simulink model "2293_2020_TP1_Parra_fgh"  (R2019b)
settings: Solver=ode45  StartTime=0.0  StopTime=10  FixedStep=0.001  RelTol=1e-3
undefined symbols (not defined in the file): A, B, C, ki, kp, L, ueq, xeq, yref
settings Model: Creator=aghersin  LastModifiedBy=rochi
settings DataIOCC: ReturnWorkspaceOutputs=off
settings DebuggingCC: ArithmeticOperatorsInVariantConditions=warning
settings SFSimCC: SimUseLocalCustomCode=off  CustomCodeUndefinedFunction=UseInterfaceOnly
settings RTWCC: RTWUseLocalCustomCode=off

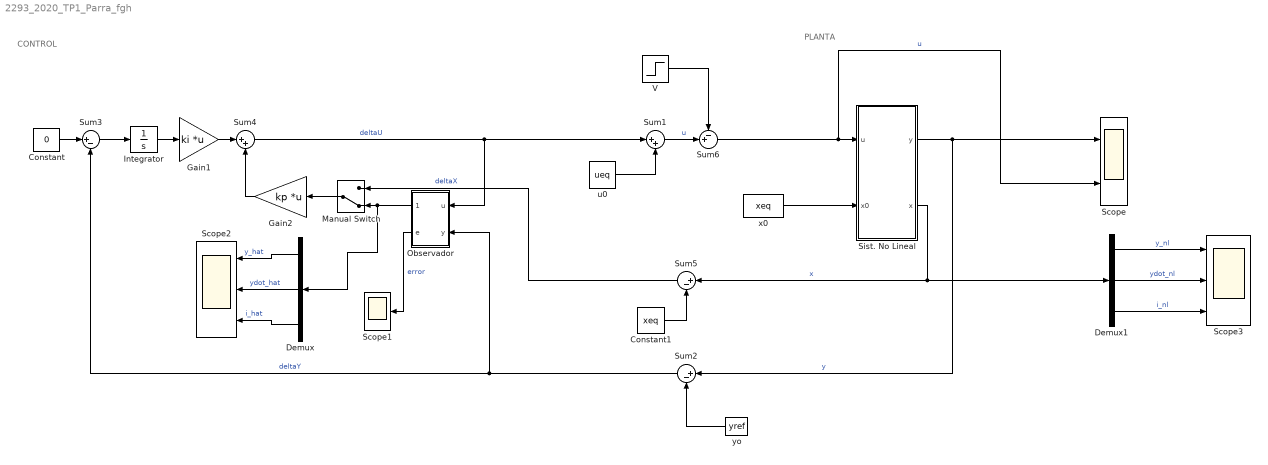
== system 2293_2020_TP1_Parra_fgh ==
  note: CONTROL
  note: PLANTA
  Constant : Constant  Value=0
  Constant1 : Constant  Value=xeq
  Demux : Demux  Outputs=3
  Demux1 : Demux  Outputs=3
  Gain1 : Gain  Gain=ki  Multiplication=Matrix(K*u)
  Gain2 : Gain  Gain=kp  Multiplication=Matrix(K*u)
  Integrator : Integrator
  Manual Switch : ManualSwitch  CurrentSetting=0
  Observador : Subsystem
  Scope : Scope  NumInputPorts=2
  Scope1 : Scope
  Scope2 : Scope  NumInputPorts=3
  Scope3 : Scope  NumInputPorts=3
  "Sist. No Lineal " : Subsystem
  Sum1 : Sum  Inputs=|++
  Sum2 : Sum  Inputs=|+-
  Sum3 : Sum  Inputs=|+-
  Sum4 : Sum  Inputs=|++
  Sum5 : Sum  Inputs=|+-
  Sum6 : Sum  Inputs=-+|
  V : Step  Time=5  SampleTime=0
  u0 : Constant  Value=ueq
  x0 : Constant  Value=xeq
  yo : Constant  Value=yref
  wires:
  Gain2/1 -> Sum4/2
  Sum4/1 -> Sum1/1, Observador/1(u)  "deltaU"
  Constant/1 -> Sum3/1
  Sum3/1 -> Integrator/1
  u0/1 -> Sum1/2
  Integrator/1 -> Gain1/1
  Sum1/1 -> Sum6/2  "u"
  Observador/2(e) -> Scope1/1  "error"
  Manual Switch/1 -> Gain2/1
  Observador/1(xhat) -> Demux/1, Manual Switch/2
  Gain1/1 -> Sum4/1
  V/1 -> Sum6/1
  Sum6/1 -> Scope/2, "Sist. No Lineal "/1(u)  "u"
  "Sist. No Lineal "/2(x) -> Demux1/1, Sum5/1  "x"
  "Sist. No Lineal "/1(y) -> Scope/1, Sum2/1  "y"
  x0/1 -> "Sist. No Lineal "/2(x0)
  yo/1 -> Sum2/2
  Sum2/1 -> Observador/2(y), Sum3/2  "deltaY"
  Sum5/1 -> Manual Switch/1  "deltaX"
  Demux/2 -> Scope2/2  "ydot_hat"
  Demux/1 -> Scope2/1  "y_hat"
  Demux/3 -> Scope2/3  "i_hat"
  Demux1/1 -> Scope3/1  "y_nl"
  Demux1/2 -> Scope3/2  "ydot_nl"
  Demux1/3 -> Scope3/3  "i_nl"
  Constant1/1 -> Sum5/2

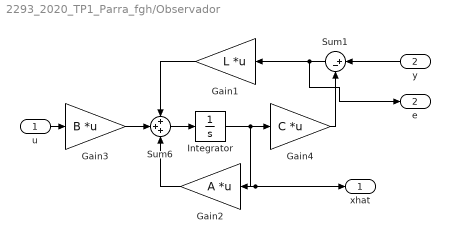
== system 2293_2020_TP1_Parra_fgh/Observador ==
  u : Inport
  y : Inport  Port=2
  Gain1 : Gain  Gain=L  Multiplication=Matrix(K*u)
  Gain2 : Gain  Gain=A  Multiplication=Matrix(K*u)
  Gain3 : Gain  Gain=B  Multiplication=Matrix(K*u)
  Gain4 : Gain  Gain=C  Multiplication=Matrix(K*u)
  Integrator : Integrator
  Sum1 : Sum  Inputs=|+-
  Sum6 : Sum  Inputs=+++
  xhat : Outport  VectorParamsAs1DForOutWhenUnconnected=off
  e : Outport  Port=2  VectorParamsAs1DForOutWhenUnconnected=off
  wires:
  Gain2/1 -> Sum6/3
  Integrator/1 -> Gain4/1, xhat/1, Gain2/1
  u/1 -> Gain3/1
  Sum6/1 -> Integrator/1
  Gain4/1 -> Sum1/2
  Gain3/1 -> Sum6/2
  Sum1/1 -> e/1, Gain1/1
  y/1 -> Sum1/1
  Gain1/1 -> Sum6/1

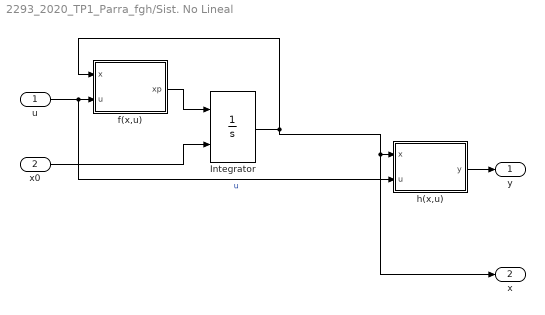
== system 2293_2020_TP1_Parra_fgh/Sist. No Lineal  ==
  u : Inport
  x0 : Inport  Port=2
  Integrator : Integrator  InitialConditionSource=external  LimitOutput=on  UpperSaturationLimit=[0.995, 500, 10]  LowerSaturationLimit=-[0.995, 500, 10]
  f(x,u) : MATLAB Function  TreatAsAtomicUnit=on
  h(x,u) : MATLAB Function  TreatAsAtomicUnit=on
  y : Outport  VectorParamsAs1DForOutWhenUnconnected=off
  x : Outport  Port=2  VectorParamsAs1DForOutWhenUnconnected=off
  wires:
  h(x,u)/1(y) -> y/1
  u/1 -> h(x,u)/2(u), f(x,u)/2(u)  "u"
  f(x,u)/1(xp) -> Integrator/1
  x0/1 -> Integrator/2
  Integrator/1 -> x/1, h(x,u)/1(x), f(x,u)/1(x)

== matlab function 2293_2020_TP1_Parra_fgh/Sist. No Lineal /f(x,u) ==
  data: x input; u input; xp output
function xp  = f(x, u)

LIMIT = 0.99;
if abs(x(1)) <= LIMIT
    xp1 = x(2);
    xp2 = (5*(x(3) + 2)^2)/(2*(x(1) - 1)^2) ...
        - (5*(x(3) - 2)^2)/(2*(x(1) + 1)^2) - 10; 
else
    xp1 = 0;
    xp2 = 0;    
end

xp3 = - 4*x(3)^2 + u;
xp = [xp1; xp2; xp3];

== matlab function 2293_2020_TP1_Parra_fgh/Sist. No Lineal /h(x,u) ==
  data: x input; u input; y output
function y = h(x,u)

y=x(1);
